simulink model "QP_Solver"  (R2015a)
settings: Solver=FixedStepDiscrete  StartTime=0.0  StopTime=0.01  FixedStep=0.01  RelTol=1e-3
values from neighbouring files (symbols this model uses):
  constraints = struct    [user_Inputs.m]
  f = [-4.2096152960; -2.8665461266]    [user_Inputs.m]
  lam_old = lam.Data    [user_Inputs.m]
  model = struct    [user_Inputs.m]
  QP = struct    [user_Inputs.m]
  U_unc = [0.0254; -0.3325]    [user_Inputs.m]
libraries: simulink x3
settings Model: Creator=vinay  LastModifiedBy=vinay

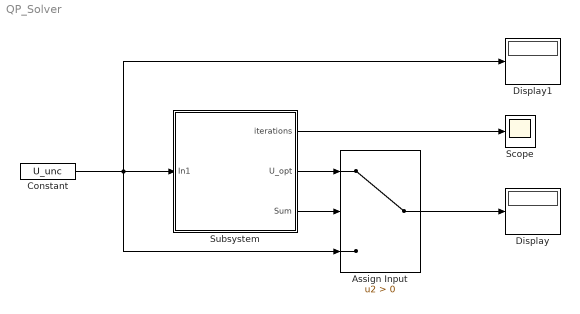
== system QP_Solver ==
  Assign Input : Switch  Criteria=u2 > Threshold
  Constant : Constant  Value=U_unc
  Display : Display
  Display1 : Display
  Scope : Scope
  Subsystem : Subsystem
      mask Display: disp('MPC\nOptimization')
  wires:
  Assign Input/1 -> Display/1
  Constant/1 -> Assign Input/3, Display1/1, Subsystem/1(In1)
  Subsystem/2(U_opt) -> Assign Input/1
  Subsystem/3(Sum) -> Assign Input/2
  Subsystem/1(iterations) -> Scope/1

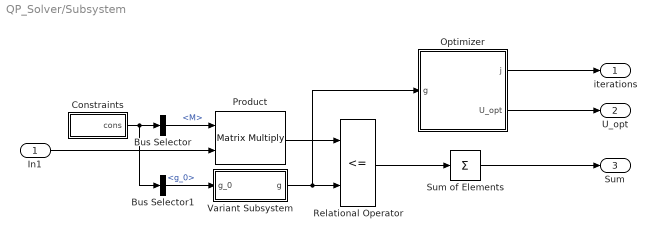
== system QP_Solver/Subsystem ==
  In1 : Inport
  Bus Selector : BusSelector  OutputSignals=M
  Bus Selector1 : BusSelector  OutputSignals=g_0
  Constraints : Subsystem
      mask Display: disp('M, g_0','texmode','on')
  Optimizer : Subsystem
      mask Display: disp('PQP\nOptimizer')
  Product : Product  Multiplication=Matrix(*)
      mask Display: disp('MU')
  Relational Operator : RelationalOperator  Operator=<=  OutDataTypeStr=boolean
  Sum of Elements : Sum  Inputs=+
  Variant Subsystem : Subsystem  Variant=on
      mask Display: disp('Format g_0','texmode','on')
  iterations : Outport
  U_opt : Outport  Port=2
  Sum : Outport  Port=3
  wires:
  Optimizer/2(U_opt) -> U_opt/1
  In1/1 -> Product/2
  Bus Selector/1 -> Product/1  "<M>"
  Product/1 -> Relational Operator/1
  Constraints/1(cons) -> Bus Selector1/1, Bus Selector/1
  Variant Subsystem/1(g) -> Optimizer/1(g), Relational Operator/2
  Sum of Elements/1 -> Sum/1
  Relational Operator/1 -> Sum of Elements/1
  Bus Selector1/1 -> Variant Subsystem/1(g_0)  "<g_0>"
  Optimizer/1(j) -> iterations/1

== system QP_Solver/Subsystem/Constraints ==
  Bus Creator : BusCreator  Inputs=2
  Constant1 : Constant  Value=constraints.M
  Constant2 : Constant  Value=constraints.g
  cons : Outport
  wires:
  Bus Creator/1 -> cons/1
  Constant1/1 -> Bus Creator/1  "M"
  Constant2/1 -> Bus Creator/2  "g_0"

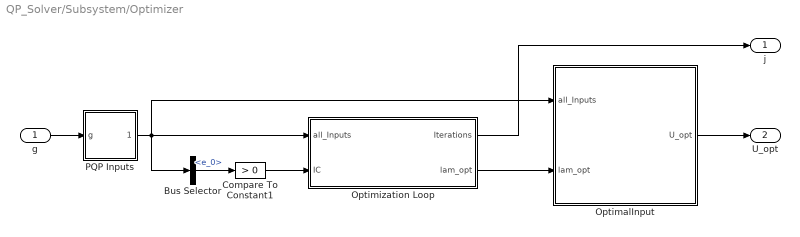
== system QP_Solver/Subsystem/Optimizer ==
  g : Inport
  Bus Selector : BusSelector  OutputSignals=PQP_in.e_0
  Compare To Constant1 : simulink/Logic and Bit Operations/Compare To Constant  relop=>  const=0  OutDataTypeStr=boolean
  OptimalInput : Subsystem
      mask Display: disp('U_{opt}=-H^{-1}(f+0.5M^T\lambda)','texmode','on')
  Optimization Loop : Subsystem  TreatAsAtomicUnit=on
  PQP Inputs : Subsystem
      mask Display: disp('PQP\nInputs')
  j : Outport
  U_opt : Outport  Port=2
  wires:
  g/1 -> PQP Inputs/1(g)
  Bus Selector/1 -> Compare To Constant1/1  "<e_0>"
  PQP Inputs/1(all_Inputs) -> OptimalInput/1(all_Inputs), Bus Selector/1, Optimization Loop/1(all_Inputs)
  Compare To Constant1/1 -> Optimization Loop/2(IC)
  Optimization Loop/2(lam_opt) -> OptimalInput/2(lam_opt)
  Optimization Loop/1(Iterations) -> j/1
  OptimalInput/1(U_opt) -> U_opt/1

== system QP_Solver/Subsystem/Variant Subsystem ==
  g_0 : Inport
  Append : Subsystem  VariantControl=g_init == 1
      mask Display: disp('g_0 \in R^x\rightarrow g \in R^{2x}', 'texmode','on')
  NoAppend : Subsystem  VariantControl=g_init == 0
      mask Display: disp('Input (g_0) = Output (g_0 = g)', 'texmode','on')
  g : Outport

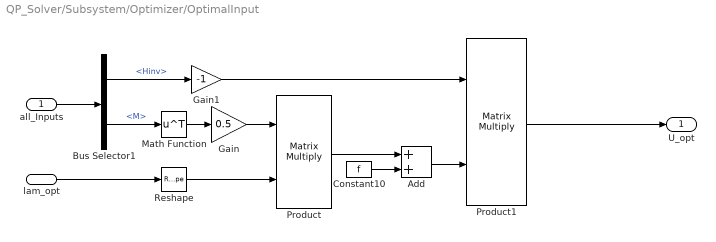
== system QP_Solver/Subsystem/Optimizer/OptimalInput ==
  all_Inputs : Inport
  lam_opt : Inport  Port=2
  Add : Sum
  Bus Selector1 : BusSelector  OutputSignals=PQP_in.Hinv,PQP_in.M
  Constant10 : Constant  Value=f
  Gain : Gain  Gain=0.5
  Gain1 : Gain  Gain=-1
  Math Function : Math  Operator=transpose  SaturateOnIntegerOverflow=on
  Product : Product  Multiplication=Matrix(*)
  Product1 : Product  Multiplication=Matrix(*)
  Reshape : Reshape  OutputDimensionality=Column vector (2-D)  OutputDimensions=[4,1]
  U_opt : Outport
  wires:
  Bus Selector1/2 -> Math Function/1  "<M>"
  Reshape/1 -> Product/2
  Math Function/1 -> Gain/1
  Bus Selector1/1 -> Gain1/1  "<Hinv>"
  lam_opt/1 -> Reshape/1
  all_Inputs/1 -> Bus Selector1/1
  Product1/1 -> U_opt/1
  Gain/1 -> Product/1
  Product/1 -> Add/1
  Add/1 -> Product1/2
  Gain1/1 -> Product1/1
  Constant10/1 -> Add/2

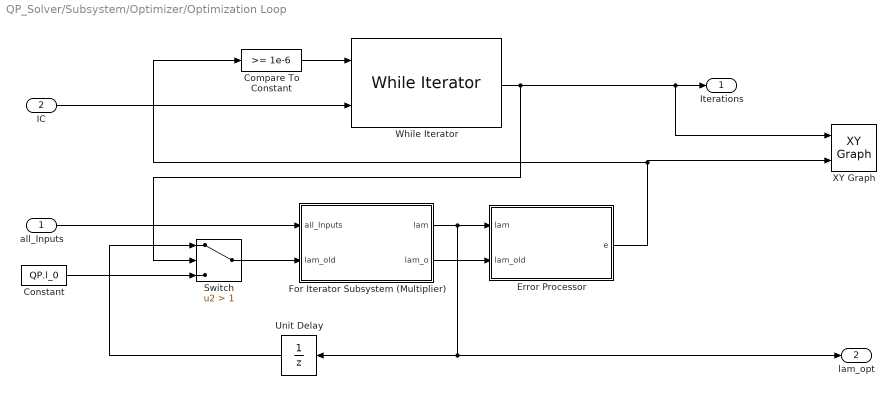
== system QP_Solver/Subsystem/Optimizer/Optimization Loop ==
  all_Inputs : Inport
  IC : Inport  Port=2
  Compare To Constant : simulink/Logic and Bit Operations/Compare To Constant  relop=>=  const=1e-6  OutDataTypeStr=boolean
  Constant : Constant  Value=QP.l_0
  Error Processor : Subsystem
      mask Display: disp('e_j=\Delta\lambda^T\Delta\lambda','texmode','on')
  For Iterator Subsystem (Multiplier) : Subsystem  TreatAsAtomicUnit=on
  Switch : Switch  Criteria=u2 > Threshold  Threshold=1
  Unit Delay : UnitDelay  InitialCondition=lam_old  SampleTime=-1
  While Iterator : WhileIterator  MaxIters=700  ResetStates=reset  ShowIterationPort=on
  XY Graph : simulink/Sinks/XY Graph  xmin=0  xmax=700  ymin=0  ymax=250  st=-1
  Iterations : Outport
  lam_opt : Outport  Port=2
  wires:
  Compare To Constant/1 -> While Iterator/1
  IC/1 -> While Iterator/2
  Error Processor/1(e) -> XY Graph/2, Compare To Constant/1
  all_Inputs/1 -> For Iterator Subsystem (Multiplier)/1(all_Inputs)
  While Iterator/1 -> Switch/2, XY Graph/1, Iterations/1
  Constant/1 -> Switch/3
  Switch/1 -> For Iterator Subsystem (Multiplier)/2(lam_old)
  Unit Delay/1 -> Switch/1
  For Iterator Subsystem (Multiplier)/2(lam_o) -> Error Processor/2(lam_old)
  For Iterator Subsystem (Multiplier)/1(lam) -> Error Processor/1(lam), lam_opt/1, Unit Delay/1

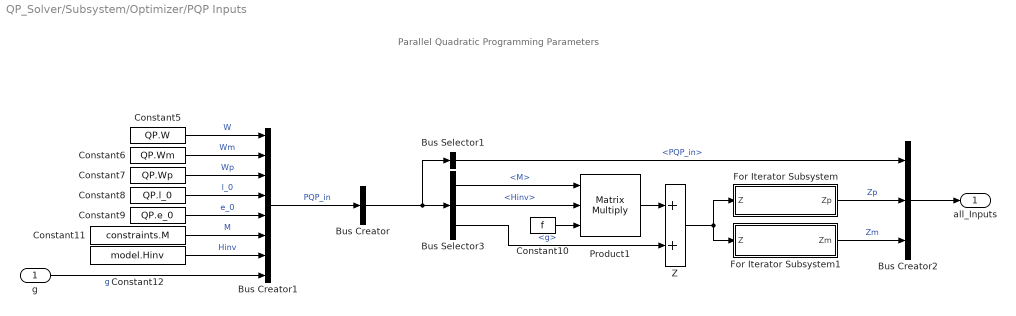
== system QP_Solver/Subsystem/Optimizer/PQP Inputs ==
  note: Parallel Quadratic Programming Parameters
  g : Inport
  Bus Creator : BusCreator  Inputs=1
  Bus Creator1 : BusCreator  Inputs=8
  Bus Creator2 : BusCreator  Inputs=3
  Bus Selector1 : BusSelector  OutputSignals=PQP_in
  Bus Selector3 : BusSelector  OutputSignals=PQP_in.M,PQP_in.Hinv,PQP_in.g
  Constant10 : Constant  Value=f
  Constant11 : Constant  Value=constraints.M
  Constant12 : Constant  Value=model.Hinv
  Constant5 : Constant  Value=QP.W
  Constant6 : Constant  Value=QP.Wm
  Constant7 : Constant  Value=QP.Wp
  Constant8 : Constant  Value=QP.l_0
  Constant9 : Constant  Value=QP.e_0
  For Iterator Subsystem : Subsystem  TreatAsAtomicUnit=on
      mask Display: disp('Z_p = max(Z,0)','texmode','on')
  For Iterator Subsystem1 : Subsystem  TreatAsAtomicUnit=on
      mask Display: disp('Z_m = max(-Z,0)','texmode','on')
  Product1 : Product  Inputs=3  Multiplication=Matrix(*)
      mask Display: disp('M[H^{-1}]f','texmode','on')
  Z : Sum
  all_Inputs : Outport
  wires:
  Bus Creator1/1 -> Bus Creator/1  "PQP_in"
  Constant5/1 -> Bus Creator1/1  "W"
  Constant11/1 -> Bus Creator1/6  "M"
  Constant9/1 -> Bus Creator1/5  "e_0"
  Constant6/1 -> Bus Creator1/2  "Wm"
  Constant7/1 -> Bus Creator1/3  "Wp"
  Constant12/1 -> Bus Creator1/7  "Hinv"
  Constant8/1 -> Bus Creator1/4  "l_0"
  g/1 -> Bus Creator1/8  "g"
  Z/1 -> For Iterator Subsystem/1(Z), For Iterator Subsystem1/1(Z)
  Constant10/1 -> Product1/3
  Bus Selector3/3 -> Z/2  "<g>"
  Bus Creator/1 -> Bus Selector1/1, Bus Selector3/1
  Bus Selector3/1 -> Product1/1  "<M>"
  Product1/1 -> Z/1
  Bus Selector3/2 -> Product1/2  "<Hinv>"
  Bus Selector1/1 -> Bus Creator2/1  "<PQP_in>"
  For Iterator Subsystem/1(Zp) -> Bus Creator2/2  "Zp"
  For Iterator Subsystem1/1(Zm) -> Bus Creator2/3  "Zm"
  Bus Creator2/1 -> all_Inputs/1

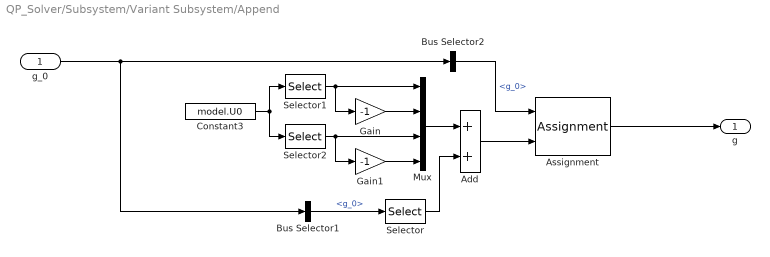
== system QP_Solver/Subsystem/Variant Subsystem/Append ==
  g_0 : Inport
  Add : Sum
  Assignment : Assignment  DiagnosticForDimensions=Warning  Indices=[5 6 7 8]
  Bus Selector1 : BusSelector  OutputSignals=g_0
  Bus Selector2 : BusSelector  OutputSignals=g_0
  Constant3 : Constant  Value=model.U0
  Gain : Gain  Gain=-1
  Gain1 : Gain  Gain=-1
  Mux : Mux
  Selector : Selector  InputPortWidth=8  Indices=[5 6 7 8]
  Selector1 : Selector  InputPortWidth=2  Indices=[1]
  Selector2 : Selector  InputPortWidth=2  Indices=[2]
  g : Outport
  wires:
  g_0/1 -> Bus Selector2/1, Bus Selector1/1
  Constant3/1 -> Selector1/1, Selector2/1
  Assignment/1 -> g/1
  Selector1/1 -> Mux/1, Gain/1
  Bus Selector1/1 -> Selector/1  "<g_0>"
  Add/1 -> Assignment/2
  Gain1/1 -> Mux/4
  Selector2/1 -> Mux/3, Gain1/1
  Gain/1 -> Mux/2
  Selector/1 -> Add/2
  Mux/1 -> Add/1
  Bus Selector2/1 -> Assignment/1  "<g_0>"

== system QP_Solver/Subsystem/Variant Subsystem/NoAppend ==
  g_0 : Inport
  g : Outport
  wires:
  g_0/1 -> g/1

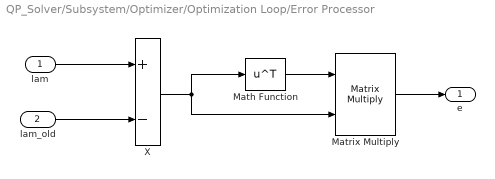
== system QP_Solver/Subsystem/Optimizer/Optimization Loop/Error Processor ==
  lam : Inport
  lam_old : Inport  Port=2
  Math Function : Math  Operator=transpose  SaturateOnIntegerOverflow=on
  Matrix Multiply : Product  Multiplication=Matrix(*)  OutDataTypeStr=double
  X : Sum  Inputs=+-
  e : Outport
  wires:
  Math Function/1 -> Matrix Multiply/1
  lam_old/1 -> X/2
  lam/1 -> X/1
  X/1 -> Math Function/1, Matrix Multiply/2
  Matrix Multiply/1 -> e/1

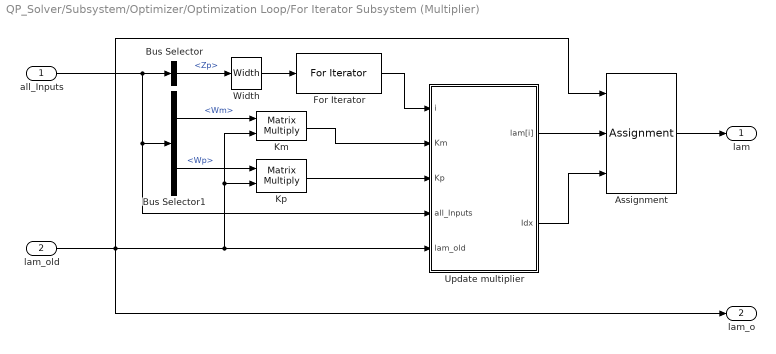
== system QP_Solver/Subsystem/Optimizer/Optimization Loop/For Iterator Subsystem (Multiplier) ==
  all_Inputs : Inport
  lam_old : Inport  Port=2
  Assignment : Assignment  DiagnosticForDimensions=Warning  IndexOptions=Index vector (port)
  Bus Selector : BusSelector  OutputSignals=Zp
  Bus Selector1 : BusSelector  OutputSignals=PQP_in.Wm,PQP_in.Wp
  For Iterator : ForIterator  IterationSource=external
  Km : Product  Multiplication=Matrix(*)
  Kp : Product  Multiplication=Matrix(*)
  Update multiplier : Subsystem
      mask Display: disp('Solve for \lambda_i','texmode','on')
  Width : Width
  lam : Outport
  lam_o : Outport  Port=2
  wires:
  all_Inputs/1 -> Update multiplier/4(all_Inputs), Bus Selector1/1, Bus Selector/1
  Bus Selector/1 -> Width/1  "<Zp>"
  Width/1 -> For Iterator/1
  Bus Selector1/1 -> Km/1  "<Wm>"
  Bus Selector1/2 -> Kp/1  "<Wp>"
  For Iterator/1 -> Update multiplier/1(i)
  Km/1 -> Update multiplier/2(Km)
  Kp/1 -> Update multiplier/3(Kp)
  Update multiplier/2(Idx) -> Assignment/3
  Update multiplier/1(lam[i]) -> Assignment/2
  lam_old/1 -> lam_o/1, Update multiplier/5(lam_old), Kp/2, Km/2, Assignment/1
  Assignment/1 -> lam/1

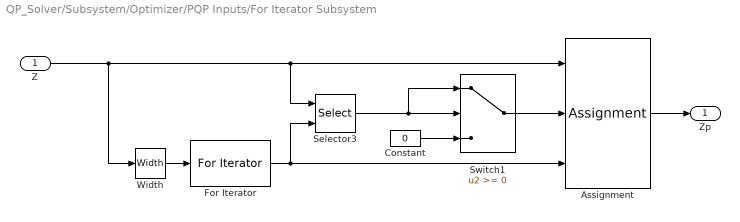
== system QP_Solver/Subsystem/Optimizer/PQP Inputs/For Iterator Subsystem ==
  Z : Inport
  Assignment : Assignment  DiagnosticForDimensions=Warning  IndexOptions=Index vector (port)
  Constant : Constant  Value=0
  For Iterator : ForIterator  IterationSource=external  IterationLimit=8
  Selector3 : Selector  InputPortWidth=4  IndexOptions=Index vector (port)  Indices=[1 3]
  Switch1 : Switch
  Width : Width  DataType=int32
  Zp : Outport
  wires:
  For Iterator/1 -> Selector3/2, Assignment/3
  Selector3/1 -> Switch1/1, Switch1/2
  Z/1 -> Assignment/1, Selector3/1, Width/1
  Width/1 -> For Iterator/1
  Switch1/1 -> Assignment/2
  Assignment/1 -> Zp/1
  Constant/1 -> Switch1/3

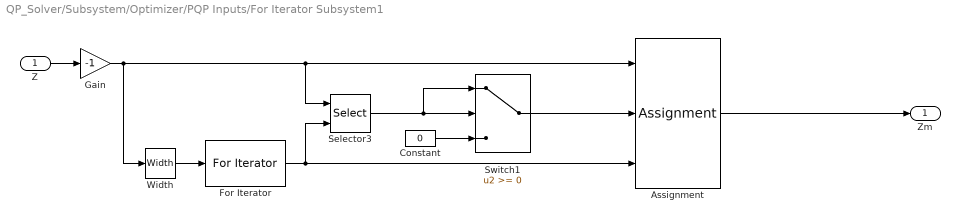
== system QP_Solver/Subsystem/Optimizer/PQP Inputs/For Iterator Subsystem1 ==
  Z : Inport
  Assignment : Assignment  DiagnosticForDimensions=Warning  IndexOptions=Index vector (port)
  Constant : Constant  Value=0
  For Iterator : ForIterator  IterationSource=external  IterationLimit=8
  Gain : Gain  Gain=-1
  Selector3 : Selector  InputPortWidth=4  IndexOptions=Index vector (port)  Indices=[1 3]
  Switch1 : Switch
  Width : Width  DataType=int32
  Zm : Outport
  wires:
  Constant/1 -> Switch1/3
  Assignment/1 -> Zm/1
  Switch1/1 -> Assignment/2
  Width/1 -> For Iterator/1
  Z/1 -> Gain/1
  Selector3/1 -> Switch1/2, Switch1/1
  For Iterator/1 -> Assignment/3, Selector3/2
  Gain/1 -> Width/1, Selector3/1, Assignment/1

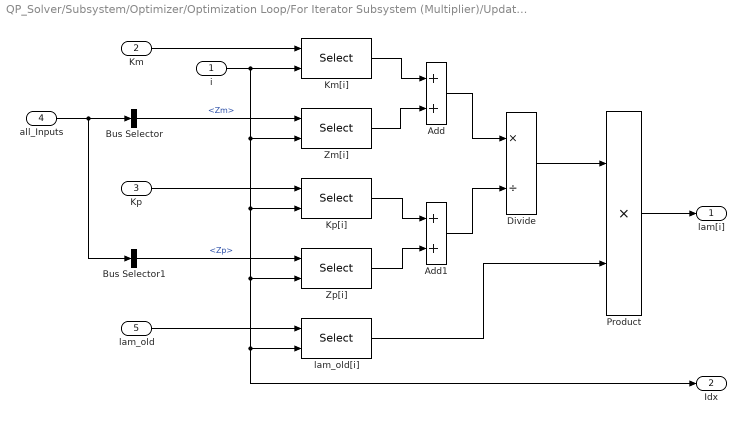
== system QP_Solver/Subsystem/Optimizer/Optimization Loop/For Iterator Subsystem (Multiplier)/Update multiplier ==
  i : Inport
  Km : Inport  Port=2
  Kp : Inport  Port=3
  all_Inputs : Inport  Port=4
  lam_old : Inport  Port=5
  Add : Sum
  Add1 : Sum
  Bus Selector : BusSelector  OutputSignals=Zm
  Bus Selector1 : BusSelector  OutputSignals=Zp
  Divide : Product  Inputs=*/
  Km[i] : Selector  InputPortWidth=4  IndexOptions=Index vector (port)  Indices=[1 3]
  Kp[i] : Selector  InputPortWidth=4  IndexOptions=Index vector (port)  Indices=[1 3]
  Product : Product
  Zm[i] : Selector  InputPortWidth=4  IndexOptions=Index vector (port)  Indices=[1 3]
  Zp[i] : Selector  InputPortWidth=4  IndexOptions=Index vector (port)  Indices=[1 3]
  lam_old[i] : Selector  InputPortWidth=4  IndexOptions=Index vector (port)  Indices=[1 3]
  lam[i] : Outport
  Idx : Outport  Port=2
  wires:
  Km/1 -> Km[i]/1
  Kp/1 -> Kp[i]/1
  lam_old/1 -> lam_old[i]/1
  all_Inputs/1 -> Bus Selector1/1, Bus Selector/1
  Bus Selector/1 -> Zm[i]/1  "<Zm>"
  Bus Selector1/1 -> Zp[i]/1  "<Zp>"
  Km[i]/1 -> Add/1
  Zm[i]/1 -> Add/2
  Kp[i]/1 -> Add1/1
  Zp[i]/1 -> Add1/2
  lam_old[i]/1 -> Product/2
  Add1/1 -> Divide/2
  Add/1 -> Divide/1
  Divide/1 -> Product/1
  Product/1 -> lam[i]/1
  i/1 -> Idx/1, lam_old[i]/2, Zp[i]/2, Kp[i]/2, Zm[i]/2, Km[i]/2
